simulink model "Laboratory_1_Independent"  (R2023b)
settings: Solver=FixedStepDiscrete  StartTime=0.0  StopTime=10.0  FixedStep=0.1  RelTol=1e-3
settings Model: Creator=cosmi  LastModifiedBy=cosmi

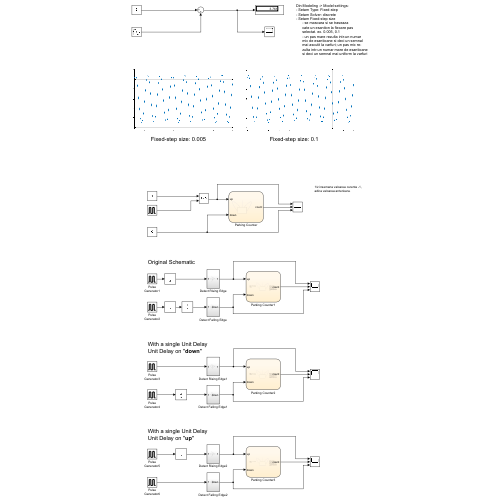
[thumbnail: Simulink's stored preview of the top-level diagram]
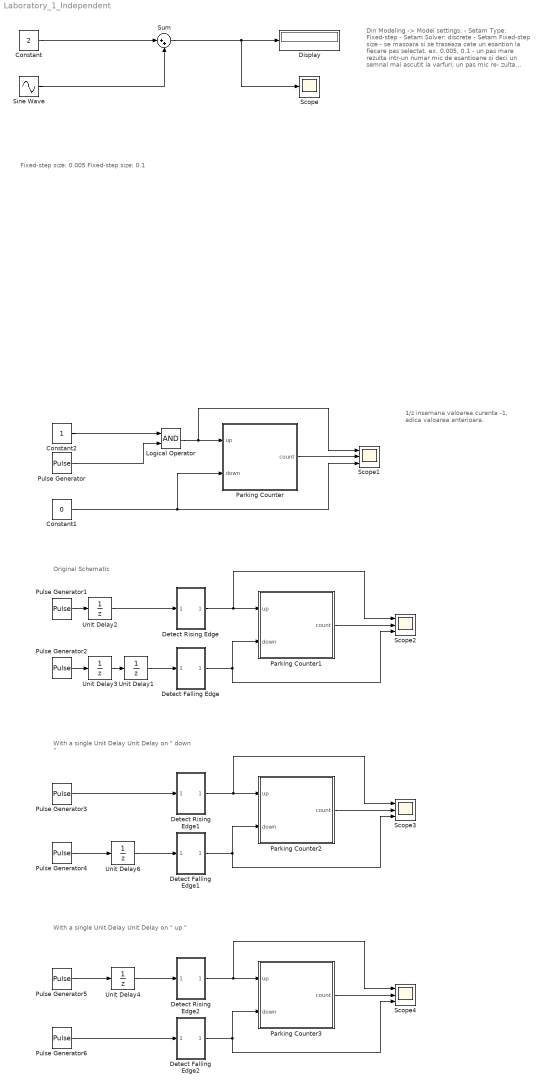
== system Laboratory_1_Independent ==
  note: With a single Unit Delay
      | Unit Delay on " down "
  note: Original Schematic
  note: 1/z insemana valoarea curenta -1,
      | adica valoarea anterioara.
  note: Fixed-step size: 0.005 Fixed-step size: 0.1
  note: Din Modeling -> Model settings:
      | - Setam Type: Fixed-step
      | - Setam Solver: discrete
      | - Setam Fixed-step size
      | - se masoara si se traseaza
      | cate un esantion la fiecare pas
      | selectat. ex. 0.005, 0.1
      | - un pas mare rezulta intr-un numar
      | mic de esantioane si deci un semnal
      | mai ascutit la varfuri; un pas mic re-
      | zulta intr-un numar mare de esantioane
      | si deci un semnal mai uniform la varfuri
  note: With a single Unit Delay
      | Unit Delay on " up "
  Constant : Constant  Value=2
  Constant1 : Constant  Value=0  OutDataTypeStr=boolean
  Constant2 : Constant
  Detect Falling Edge : Subsystem
  Detect Falling Edge1 : Subsystem
  Detect Falling Edge2 : Subsystem
  Detect Rising Edge : Subsystem
  Detect Rising Edge1 : Subsystem
  Detect Rising Edge2 : Subsystem
  Display : Display
  Logical Operator : Logic  AllPortsSameDT=off  OutDataTypeStr=boolean
  Parking Counter : Stateflow chart  TreatAsAtomicUnit=on
      settings: PortSchema="{\"entries\":[{\"content\":{\"sides\":[{\"content\":{\"connectorIds\":[\"In2\",\"In1\"]},\"type\":\"ConnectorPlacement.EquallySpacedRectSide\",\"uuid\":\"8102f69c-6126-4e4c-ad27-47c4370921f8\"},{\"content\":{\"connectorIds\":[\"Out1\"],\"side\":\"RIGHT\"},\"type\":\"ConnectorPlacement.EquallySpacedRectSide\",\"uuid\":\"6278366f-aa8b-48e0-b55e-8a4805962828\"},{\"content\":{\"side\":\"TOP\"},\"type\":\"ConnectorPlacement.EquallySpacedRectSide\",\"uuid\":\"04b958e9-0f20-4a5b-bf35-4e2d9e4d9da2\"}]},\"type\":\"ConnectorPlacement.EquallySpacedConnector\",\"uuid\":\"f38d4fe2-86ec-457f-b9ee-3c6784020d1b\"}],\"packageUris\":[\"http://schema.mathworks.com/mf0/Connector/R2020b\"],\"version\":\"1.0\"}"
  Parking Counter1 : Stateflow chart  TreatAsAtomicUnit=on
      settings: PortSchema="{\"entries\":[{\"content\":{\"sides\":[{\"content\":{\"connectorIds\":[\"In2\",\"In1\"]},\"type\":\"ConnectorPlacement.EquallySpacedRectSide\",\"uuid\":\"8102f69c-6126-4e4c-ad27-47c4370921f8\"},{\"content\":{\"connectorIds\":[\"Out1\"],\"side\":\"RIGHT\"},\"type\":\"ConnectorPlacement.EquallySpacedRectSide\",\"uuid\":\"6278366f-aa8b-48e0-b55e-8a4805962828\"},{\"content\":{\"side\":\"TOP\"},\"type\":\"ConnectorPlacement.EquallySpacedRectSide\",\"uuid\":\"04b958e9-0f20-4a5b-bf35-4e2d9e4d9da2\"}]},\"type\":\"ConnectorPlacement.EquallySpacedConnector\",\"uuid\":\"f38d4fe2-86ec-457f-b9ee-3c6784020d1b\"}],\"packageUris\":[\"http://schema.mathworks.com/mf0/Connector/R2020b\"],\"version\":\"1.0\"}"
  Parking Counter2 : Stateflow chart  TreatAsAtomicUnit=on
      settings: PortSchema="{\"entries\":[{\"content\":{\"sides\":[{\"content\":{\"connectorIds\":[\"In2\",\"In1\"]},\"type\":\"ConnectorPlacement.EquallySpacedRectSide\",\"uuid\":\"8102f69c-6126-4e4c-ad27-47c4370921f8\"},{\"content\":{\"connectorIds\":[\"Out1\"],\"side\":\"RIGHT\"},\"type\":\"ConnectorPlacement.EquallySpacedRectSide\",\"uuid\":\"6278366f-aa8b-48e0-b55e-8a4805962828\"},{\"content\":{\"side\":\"TOP\"},\"type\":\"ConnectorPlacement.EquallySpacedRectSide\",\"uuid\":\"04b958e9-0f20-4a5b-bf35-4e2d9e4d9da2\"}]},\"type\":\"ConnectorPlacement.EquallySpacedConnector\",\"uuid\":\"f38d4fe2-86ec-457f-b9ee-3c6784020d1b\"}],\"packageUris\":[\"http://schema.mathworks.com/mf0/Connector/R2020b\"],\"version\":\"1.0\"}"
  Parking Counter3 : Stateflow chart  TreatAsAtomicUnit=on
      settings: PortSchema="{\"entries\":[{\"content\":{\"sides\":[{\"content\":{\"connectorIds\":[\"In2\",\"In1\"]},\"type\":\"ConnectorPlacement.EquallySpacedRectSide\",\"uuid\":\"8102f69c-6126-4e4c-ad27-47c4370921f8\"},{\"content\":{\"connectorIds\":[\"Out1\"],\"side\":\"RIGHT\"},\"type\":\"ConnectorPlacement.EquallySpacedRectSide\",\"uuid\":\"6278366f-aa8b-48e0-b55e-8a4805962828\"},{\"content\":{\"side\":\"TOP\"},\"type\":\"ConnectorPlacement.EquallySpacedRectSide\",\"uuid\":\"04b958e9-0f20-4a5b-bf35-4e2d9e4d9da2\"}]},\"type\":\"ConnectorPlacement.EquallySpacedConnector\",\"uuid\":\"f38d4fe2-86ec-457f-b9ee-3c6784020d1b\"}],\"packageUris\":[\"http://schema.mathworks.com/mf0/Connector/R2020b\"],\"version\":\"1.0\"}"
  Pulse Generator{,1..6} (7 alike) : DiscretePulseGenerator  PulseType=Time based  Period=4  PulseWidth=10
  Scope : Scope
  Scope{1..4} (4 alike) : Scope  NumInputPorts=3
  Sine Wave : Sin  Amplitude=2.5  Frequency=5  Phase=pi/3  SampleTime=0
  Sum : Sum  Inputs=|++
  Unit Delay{1..4,6} (5 alike) : UnitDelay  SampleTime=-1  HasFrameUpgradeWarning=on
  wires:
  Constant/1 -> Sum/1
  Sine Wave/1 -> Sum/2
  Sum/1 -> Scope/1, Display/1
  Constant2/1 -> Logical Operator/1
  Pulse Generator/1 -> Logical Operator/2
  Logical Operator/1 -> Scope1/1, Parking Counter/2(up)
  Constant1/1 -> Scope1/3, Parking Counter/1(down)
  Parking Counter/1(count) -> Scope1/2
  Parking Counter1/1(count) -> Scope2/2
  Detect Rising Edge/1(Out1) -> Scope2/1, Parking Counter1/2(up)
  Detect Falling Edge/1(down) -> Scope2/3, Parking Counter1/1(down)
  Unit Delay1/1 -> Detect Falling Edge/1(In1)
  Pulse Generator1/1 -> Unit Delay2/1
  Unit Delay2/1 -> Detect Rising Edge/1(In1)
  Pulse Generator2/1 -> Unit Delay3/1
  Unit Delay3/1 -> Unit Delay1/1
  Pulse Generator4/1 -> Unit Delay6/1
  Pulse Generator3/1 -> Detect Rising Edge1/1(In1)
  Unit Delay6/1 -> Detect Falling Edge1/1(In1)
  Detect Rising Edge1/1(Out1) -> Scope3/1, Parking Counter2/2(up)
  Detect Falling Edge1/1(down) -> Scope3/3, Parking Counter2/1(down)
  Parking Counter2/1(count) -> Scope3/2
  Parking Counter3/1(count) -> Scope4/2
  Detect Falling Edge2/1(down) -> Scope4/3, Parking Counter3/1(down)
  Detect Rising Edge2/1(Out1) -> Scope4/1, Parking Counter3/2(up)
  Unit Delay4/1 -> Detect Rising Edge2/1(In1)
  Pulse Generator5/1 -> Unit Delay4/1
  Pulse Generator6/1 -> Detect Falling Edge2/1(In1)

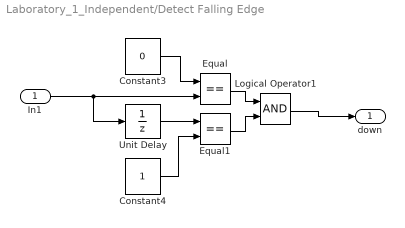
== system Laboratory_1_Independent/Detect Falling Edge ==
  In1 : Inport
  Constant3 : Constant  Value=0
  Constant4 : Constant
  Equal : RelationalOperator  Operator===  OutDataTypeStr=boolean  RndMeth=Simplest  InputSameDT=off
  Equal1 : RelationalOperator  Operator===  OutDataTypeStr=boolean  RndMeth=Simplest  InputSameDT=off
  Logical Operator1 : Logic  AllPortsSameDT=off  OutDataTypeStr=boolean
  Unit Delay : UnitDelay  SampleTime=-1  HasFrameUpgradeWarning=on
  down : Outport
  wires:
  Unit Delay/1 -> Equal1/1
  Constant3/1 -> Equal/1
  Equal/1 -> Logical Operator1/1
  In1/1 -> Unit Delay/1, Equal/2
  Logical Operator1/1 -> down/1
  Equal1/1 -> Logical Operator1/2
  Constant4/1 -> Equal1/2

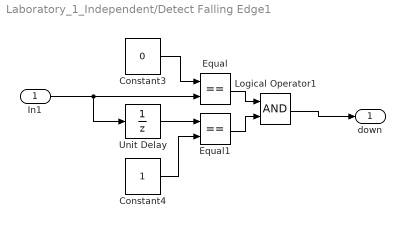
== system Laboratory_1_Independent/Detect Falling Edge1 ==
  In1 : Inport
  Constant3 : Constant  Value=0
  Constant4 : Constant
  Equal : RelationalOperator  Operator===  OutDataTypeStr=boolean  RndMeth=Simplest  InputSameDT=off
  Equal1 : RelationalOperator  Operator===  OutDataTypeStr=boolean  RndMeth=Simplest  InputSameDT=off
  Logical Operator1 : Logic  AllPortsSameDT=off  OutDataTypeStr=boolean
  Unit Delay : UnitDelay  SampleTime=-1  HasFrameUpgradeWarning=on
  down : Outport
  wires:
  Unit Delay/1 -> Equal1/1
  Constant3/1 -> Equal/1
  Equal/1 -> Logical Operator1/1
  In1/1 -> Unit Delay/1, Equal/2
  Logical Operator1/1 -> down/1
  Equal1/1 -> Logical Operator1/2
  Constant4/1 -> Equal1/2

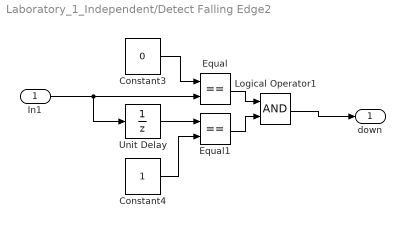
== system Laboratory_1_Independent/Detect Falling Edge2 ==
  In1 : Inport
  Constant3 : Constant  Value=0
  Constant4 : Constant
  Equal : RelationalOperator  Operator===  OutDataTypeStr=boolean  RndMeth=Simplest  InputSameDT=off
  Equal1 : RelationalOperator  Operator===  OutDataTypeStr=boolean  RndMeth=Simplest  InputSameDT=off
  Logical Operator1 : Logic  AllPortsSameDT=off  OutDataTypeStr=boolean
  Unit Delay : UnitDelay  SampleTime=-1  HasFrameUpgradeWarning=on
  down : Outport
  wires:
  Unit Delay/1 -> Equal1/1
  Constant3/1 -> Equal/1
  Equal/1 -> Logical Operator1/1
  In1/1 -> Unit Delay/1, Equal/2
  Logical Operator1/1 -> down/1
  Equal1/1 -> Logical Operator1/2
  Constant4/1 -> Equal1/2

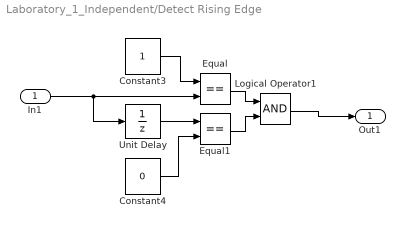
== system Laboratory_1_Independent/Detect Rising Edge ==
  In1 : Inport
  Constant3 : Constant
  Constant4 : Constant  Value=0
  Equal : RelationalOperator  Operator===  OutDataTypeStr=boolean  RndMeth=Simplest  InputSameDT=off
  Equal1 : RelationalOperator  Operator===  OutDataTypeStr=boolean  RndMeth=Simplest  InputSameDT=off
  Logical Operator1 : Logic  AllPortsSameDT=off  OutDataTypeStr=boolean
  Unit Delay : UnitDelay  SampleTime=-1  HasFrameUpgradeWarning=on
  Out1 : Outport
  wires:
  Unit Delay/1 -> Equal1/1
  Constant3/1 -> Equal/1
  Equal/1 -> Logical Operator1/1
  In1/1 -> Unit Delay/1, Equal/2
  Logical Operator1/1 -> Out1/1
  Equal1/1 -> Logical Operator1/2
  Constant4/1 -> Equal1/2

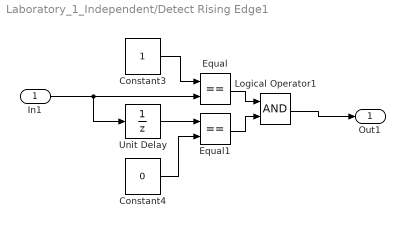
== system Laboratory_1_Independent/Detect Rising Edge1 ==
  In1 : Inport
  Constant3 : Constant
  Constant4 : Constant  Value=0
  Equal : RelationalOperator  Operator===  OutDataTypeStr=boolean  RndMeth=Simplest  InputSameDT=off
  Equal1 : RelationalOperator  Operator===  OutDataTypeStr=boolean  RndMeth=Simplest  InputSameDT=off
  Logical Operator1 : Logic  AllPortsSameDT=off  OutDataTypeStr=boolean
  Unit Delay : UnitDelay  SampleTime=-1  HasFrameUpgradeWarning=on
  Out1 : Outport
  wires:
  Unit Delay/1 -> Equal1/1
  Constant3/1 -> Equal/1
  Equal/1 -> Logical Operator1/1
  In1/1 -> Unit Delay/1, Equal/2
  Logical Operator1/1 -> Out1/1
  Equal1/1 -> Logical Operator1/2
  Constant4/1 -> Equal1/2

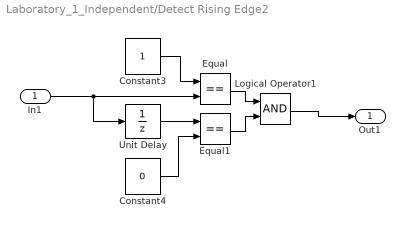
== system Laboratory_1_Independent/Detect Rising Edge2 ==
  In1 : Inport
  Constant3 : Constant
  Constant4 : Constant  Value=0
  Equal : RelationalOperator  Operator===  OutDataTypeStr=boolean  RndMeth=Simplest  InputSameDT=off
  Equal1 : RelationalOperator  Operator===  OutDataTypeStr=boolean  RndMeth=Simplest  InputSameDT=off
  Logical Operator1 : Logic  AllPortsSameDT=off  OutDataTypeStr=boolean
  Unit Delay : UnitDelay  SampleTime=-1  HasFrameUpgradeWarning=on
  Out1 : Outport
  wires:
  Unit Delay/1 -> Equal1/1
  Constant3/1 -> Equal/1
  Equal/1 -> Logical Operator1/1
  In1/1 -> Unit Delay/1, Equal/2
  Logical Operator1/1 -> Out1/1
  Equal1/1 -> Logical Operator1/2
  Constant4/1 -> Equal1/2

== stateflow chart Laboratory_1_Independent/Parking Counter1 ==
  note: Pe bara din mijloc au loc initializarile variabilelor.
      | ex: count = 0 => count este initializata
      | cu valoarea 0
  note: Din Modeling -> Model Explorer:
      | - Parking Counter:
      | - putem modifica tipul variabilelor ale FSM,
      | adica daca sa fie variabile de intrare/iesire,
      | sau daca sa fie variabile de tip int/boolean/
      | double/string/etc; deasemenea, de aici se
      | declara si variabilele folosite.
      | - inherit: same as simulink: daca selectam
      | asta, lasam defapt programul sa ghiceasca
      | ce tip de date este nevoie pentru aplicatia
      | noastra.
  state ParkingState
  (default) -> ParkingState : {count = 0;}
  ParkingState -> ParkingState [order 2] : [(up==false && down==true && count>0)]/
      | {count = count -1;}
  ParkingState -> ParkingState [order 1] : [(up==true && down==false && count<10)]/
      | {count = count +1;}
  data: down input boolean; up input boolean; count output

== stateflow chart Laboratory_1_Independent/Parking Counter2 ==
  note: Pe bara din mijloc au loc initializarile variabilelor.
      | ex: count = 0 => count este initializata
      | cu valoarea 0
  note: Din Modeling -> Model Explorer:
      | - Parking Counter:
      | - putem modifica tipul variabilelor ale FSM,
      | adica daca sa fie variabile de intrare/iesire,
      | sau daca sa fie variabile de tip int/boolean/
      | double/string/etc; deasemenea, de aici se
      | declara si variabilele folosite.
      | - inherit: same as simulink: daca selectam
      | asta, lasam defapt programul sa ghiceasca
      | ce tip de date este nevoie pentru aplicatia
      | noastra.
  state ParkingState
  (default) -> ParkingState : {count = 0;}
  ParkingState -> ParkingState [order 2] : [(up==false && down==true && count>0)]/
      | {count = count -1;}
  ParkingState -> ParkingState [order 1] : [(up==true && down==false && count<10)]/
      | {count = count +1;}
  data: down input boolean; up input boolean; count output

== stateflow chart Laboratory_1_Independent/Parking Counter ==
  state ParkingState
  (default) -> ParkingState : {count = 0;}
  ParkingState -> ParkingState [order 2] : [(up==false && down==true && count>0)]/
      | {count = count -1;}
  ParkingState -> ParkingState [order 1] : [(up==true && down==false && count<10)]/
      | {count = count +1;}
  data: down input boolean; up input boolean; count output

== stateflow chart Laboratory_1_Independent/Parking Counter3 ==
  note: Pe bara din mijloc au loc initializarile variabilelor.
      | ex: count = 0 => count este initializata
      | cu valoarea 0
  note: Din Modeling -> Model Explorer:
      | - Parking Counter:
      | - putem modifica tipul variabilelor ale FSM,
      | adica daca sa fie variabile de intrare/iesire,
      | sau daca sa fie variabile de tip int/boolean/
      | double/string/etc; deasemenea, de aici se
      | declara si variabilele folosite.
      | - inherit: same as simulink: daca selectam
      | asta, lasam defapt programul sa ghiceasca
      | ce tip de date este nevoie pentru aplicatia
      | noastra.
  state ParkingState
  (default) -> ParkingState : {count = 0;}
  ParkingState -> ParkingState [order 2] : [(up==false && down==true && count>0)]/
      | {count = count -1;}
  ParkingState -> ParkingState [order 1] : [(up==true && down==false && count<10)]/
      | {count = count +1;}
  data: down input boolean; up input boolean; count output
